simulink model "MOIsolatedBuck2"  (R2013a)
settings: Solver=ode45  StartTime=0.0  StopTime=0.25  RelTol=1e-3
libraries: powerlib x27
settings Model: Creator=Sony  LastModifiedBy=Yooshaa

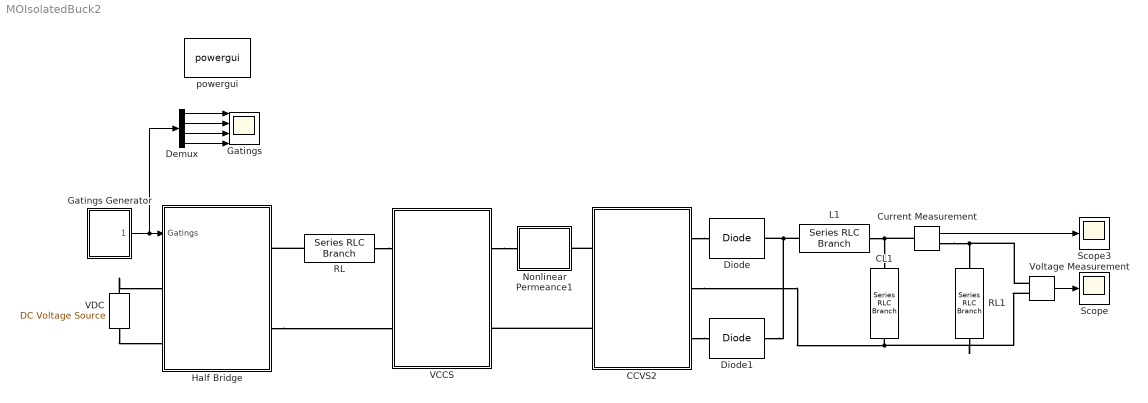
== system MOIsolatedBuck2 ==
  CCVS2 : Subsystem  mask{N=1}
  CL1 : powerlib/Elements/Series RLC Branch  LConnTagsString=__new0  RConnTagsString=__new0  BranchType=C  Resistance=1  Inductance=1e-3  SetiL0=off  InitialCurrent=0  Capacitance=1e-9  Setx0=off  InitialVoltage=0  Measurements=None
  Current Measurement : powerlib/Measurements/Current Measurement  PhasorSimulation=off  OutputType=Complex  PSBequivalent=0
  Demux : Demux
  Diode : powerlib/Power Electronics/Diode  Ron=1e-3  Lon=0  Vf=2  IC=0  UseSnubber=off  Rs=500  Cs=250e-9  Measurements=off
  Diode1 : powerlib/Power Electronics/Diode  Ron=1e-3  Lon=0  Vf=2  IC=0  UseSnubber=off  Rs=500  Cs=250e-9  Measurements=off
  Gatings : Scope  NumInputPorts=4
      settings: YMin=-1~-1~-1~-1  YMax=2~2~2~2  SaveName=ScopeData2
  Gatings Generator : Subsystem  mask{Fs=150000, D=75}
  Half Bridge : Subsystem
  L1 : powerlib/Elements/Series RLC Branch  LConnTagsString=__new0  RConnTagsString=__new0  BranchType=L  Resistance=1  Inductance=.17e-5  SetiL0=off  InitialCurrent=0  Capacitance=1e-6  Setx0=off  InitialVoltage=0  Measurements=None
  Nonlinear Permeance1 : Subsystem  mask{R=1e9, C=3.8e-5, Rm=8}
  RL : powerlib/Elements/Series RLC Branch  LConnTagsString=__new0  RConnTagsString=__new0  BranchType=RL  Resistance=1  Inductance=1e-5  SetiL0=off  InitialCurrent=0  Capacitance=1e-6  Setx0=off  InitialVoltage=0  Measurements=None
  RL1 : powerlib/Elements/Series RLC Branch  LConnTagsString=__new0  RConnTagsString=__new0  BranchType=R  Resistance=1/20  Inductance=1e-3  SetiL0=off  InitialCurrent=0  Capacitance=1e-6  Setx0=off  InitialVoltage=0  Measurements=None
  Scope : Scope
      settings: YMin=4.675  YMax=5.175  SaveName=Vou
  Scope3 : Scope
      settings: YMin=45  YMax=105  SaveName=Iou
  VCCS : Subsystem  mask{N=22}
  VDC : powerlib/Electrical Sources/DC Voltage Source  Amplitude=160  Measurements=None
  Voltage Measurement : powerlib/Measurements/Voltage Measurement  PhasorSimulation=off  OutputType=Complex  PSBequivalent=0
  powergui : powerlib/powergui  Priority=1  SimulationMode=Discrete  SolverType=Backward Euler  SampleTime=1e-7  frequency=60  SPID=on  DisableSnubberDevices=off  DisableRonSwitches=off  DisableVfSwitches=off  SwTol=0  Interpol=off  DisplayEquations=off  frequencyindice=0  Pbase=100e6  ErrMax=1e-4  Iterations=50  UnitsV=kV  UnitsW=MW  FunctionMessages=off  echomessages=off  HookPort=off  EnableUseOfTLC=off  x0status=blocks  RestoreLinks=warning  ResistiveCurrentMeasurement=off  Frange=[0:2:500]  Ylog=off  Xlog=on  ShowGrid=off  save=off  variable=ZData  ZoomFFT=off  StartTime=0.0  cycles=1  DisplayStyle=1  fundamental=60  FreqAxis=off  MaxFrequency=1000  frequencyindicesteady=1  RmsSteady=1  display=off  Ts=0  methode=off
  wires:
  Gatings Generator/1(Gatings) -> Demux/1, Half Bridge/1(Gatings)
  Voltage Measurement/1 -> Scope/1
  Current Measurement/1 -> Scope3/1
  Demux/1 -> Gatings/1
  Demux/2 -> Gatings/2
  Demux/3 -> Gatings/3
  Demux/4 -> Gatings/4
  connections:
  VDC/RConn1 -- Half Bridge/LConn1
  VDC/LConn1 -- Half Bridge/LConn2
  RL/LConn1 -- Half Bridge/RConn1
  Half Bridge/RConn2 -- VCCS/LConn2
  CCVS2/RConn1 -- Diode/LConn1
  CCVS2/RConn3 -- Diode1/LConn1
  CCVS2/RConn2 -- Voltage Measurement/LConn2 -- RL1/LConn1 -- CL1/LConn1
  VCCS/RConn1 -- Nonlinear Permeance1/LConn1
  Diode1/RConn1 -- L1/RConn1 -- Diode/RConn1
  Voltage Measurement/LConn1 -- Current Measurement/RConn1 -- RL1/RConn1
  RL/RConn1 -- VCCS/LConn1
  CCVS2/LConn1 -- Nonlinear Permeance1/RConn1
  Current Measurement/LConn1 -- L1/LConn1 -- CL1/RConn1
  CCVS2/LConn2 -- VCCS/RConn2

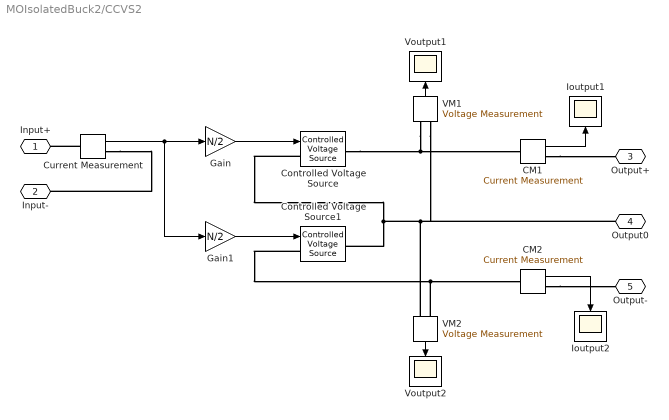
== system MOIsolatedBuck2/CCVS2 ==
  CM1 : powerlib/Measurements/Current Measurement  PhasorSimulation=off  OutputType=Complex  PSBequivalent=0
  CM2 : powerlib/Measurements/Current Measurement  PhasorSimulation=off  OutputType=Complex  PSBequivalent=0
  Controlled Voltage Source : powerlib/Electrical Sources/Controlled Voltage Source  Initialize=on  Source_Type=AC  Amplitude=0  Phase=0  Frequency=0  Measurements=None
  Controlled Voltage Source1 : powerlib/Electrical Sources/Controlled Voltage Source  Initialize=on  Source_Type=AC  Amplitude=0  Phase=0  Frequency=0  Measurements=None
  Current Measurement : powerlib/Measurements/Current Measurement  PhasorSimulation=off  OutputType=Complex  PSBequivalent=0
  Gain : Gain  Gain=N/2
  Gain1 : Gain  Gain=N/2
  Ioutput1 : Scope
      settings: YMin=-2e+10  YMax=2e+10  SaveName=Ioup
  Ioutput2 : Scope
      settings: YMin=-10  YMax=150  SaveName=Ioun
  VM1 : powerlib/Measurements/Voltage Measurement  PhasorSimulation=off  OutputType=Complex  PSBequivalent=0
  VM2 : powerlib/Measurements/Voltage Measurement  PhasorSimulation=off  OutputType=Complex  PSBequivalent=0
  Voutput1 : Scope
      settings: YMin=-2.25e+11  YMax=2.25e+11  SaveName=Voup
  Voutput2 : Scope
      settings: YMin=-20  YMax=20  SaveName=Voun
  Input+ : PMIOPort  Port=1  Side=Left
  Input- : PMIOPort  Port=2  Side=Left
  Output+ : PMIOPort  Port=3  Side=Right
  Output0 : PMIOPort  Port=4  Side=Right
  Output- : PMIOPort  Port=5  Side=Right
  wires:
  Gain/1 -> Controlled Voltage Source/1
  Current Measurement/1 -> Gain1/1, Gain/1
  Gain1/1 -> Controlled Voltage Source1/1
  VM2/1 -> Voutput2/1
  VM1/1 -> Voutput1/1
  CM2/1 -> Ioutput2/1
  CM1/1 -> Ioutput1/1
  connections:
  Current Measurement/LConn1 -- Input+/RConn1
  Current Measurement/RConn1 -- Input-/RConn1
  Controlled Voltage Source/RConn1 -- CM1/LConn1 -- VM1/LConn1
  Controlled Voltage Source/LConn1 -- Output0/RConn1 -- VM1/LConn2 -- VM2/LConn1 -- Controlled Voltage Source1/RConn1
  Controlled Voltage Source1/LConn1 -- VM2/LConn2 -- CM2/LConn1
  CM1/RConn1 -- Output+/RConn1
  CM2/RConn1 -- Output-/RConn1

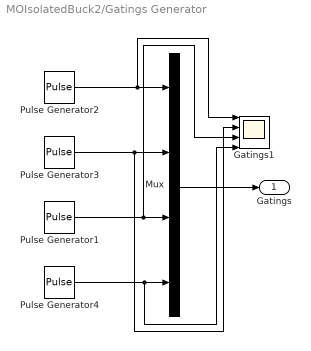
== system MOIsolatedBuck2/Gatings Generator ==
  Gatings1 : Scope  NumInputPorts=4
      settings: YMin=-1~-1~-1~-1  YMax=2~2~2~2  SaveName=ScopeData3
  Mux : Mux
  Pulse Generator1 : DiscretePulseGenerator  PulseType=Time based  Period=2/Fs  PulseWidth=50  PhaseDelay=(1/Fs)
  Pulse Generator2 : DiscretePulseGenerator  PulseType=Time based  Period=2/Fs  PulseWidth=50  PhaseDelay=-((100-D)/100)*(1/Fs)
  Pulse Generator3 : DiscretePulseGenerator  PulseType=Time based  Period=2/Fs  PulseWidth=50  PhaseDelay=(D/100)*(1/Fs)
  Pulse Generator4 : DiscretePulseGenerator  PulseType=Time based  Period=2/Fs  PulseWidth=50
  Gatings : Outport
  wires:
  Mux/1 -> Gatings/1
  Pulse Generator2/1 -> Gatings1/1, Mux/1
  Pulse Generator1/1 -> Gatings1/3, Mux/3
  Pulse Generator3/1 -> Gatings1/2, Mux/2
  Pulse Generator4/1 -> Gatings1/4, Mux/4

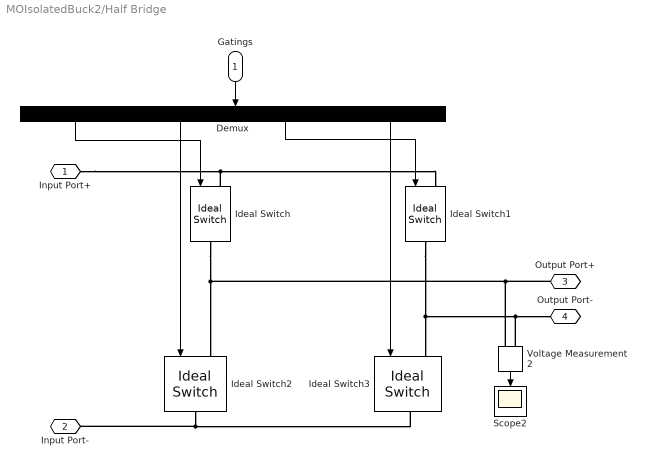
== system MOIsolatedBuck2/Half Bridge ==
  Gatings : Inport
  Demux : Demux
  Ideal Switch{,1..3} (4 alike) : powerlib/Power Electronics/Ideal Switch  Ron=0.001  Lon=0  IC=0  Rs=1e5  Cs=inf  Measurements=off
  Scope2 : Scope
      settings: YMin=-175  YMax=175  SaveName=Vinput
  Voltage Measurement2 : powerlib/Measurements/Voltage Measurement  PhasorSimulation=off  OutputType=Complex  PSBequivalent=0
  Input Port+ : PMIOPort  Port=1  Side=Left
  Input Port- : PMIOPort  Port=2  Side=Left
  Output Port+ : PMIOPort  Port=3  Side=Right
  Output Port- : PMIOPort  Port=4  Side=Right
  wires:
  Demux/3 -> Ideal Switch1/1
  Demux/1 -> Ideal Switch/1
  Demux/2 -> Ideal Switch2/1
  Gatings/1 -> Demux/1
  Demux/4 -> Ideal Switch3/1
  Voltage Measurement2/1 -> Scope2/1
  connections:
  Ideal Switch/LConn1 -- Ideal Switch1/LConn1 -- Input Port+/RConn1
  Ideal Switch2/RConn1 -- Ideal Switch3/RConn1 -- Input Port-/RConn1
  Ideal Switch1/RConn1 -- Ideal Switch3/LConn1 -- Voltage Measurement2/LConn2 -- Output Port-/RConn1
  Ideal Switch/RConn1 -- Voltage Measurement2/LConn1 -- Output Port+/RConn1 -- Ideal Switch2/LConn1

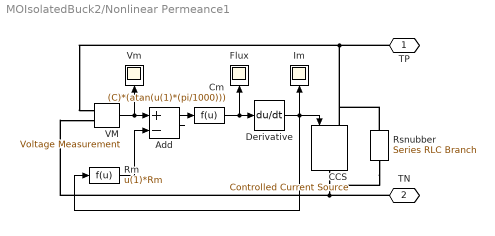
== system MOIsolatedBuck2/Nonlinear Permeance1 ==
  Add : Sum  Inputs=+-
  CCS : powerlib/Electrical Sources/Controlled Current Source  Initialize=on  Source_Type=AC  Amplitude=0  Phase=0  Frequency=0  Measurements=None
  Cm : Fcn  Expr=(C)*(atan(u(1)*(pi/1000)))
  Derivative : Derivative
  Flux : Scope
      settings: YMin=-4e-05  YMax=4e-05  SaveName=PermeanceFlux
  Im : Scope
      settings: TimeRange=0.02  YMin=-200  YMax=200  SaveName=PermeanceIm
  Rm : Fcn  Expr=u(1)*Rm
  Rsnubber : powerlib/Elements/Series RLC Branch  LConnTagsString=__new0  RConnTagsString=__new0  BranchType=R  Resistance=R  Inductance=1e-3  SetiL0=off  InitialCurrent=0  Capacitance=1e-6  Setx0=off  InitialVoltage=0  Measurements=None
  VM : powerlib/Measurements/Voltage Measurement  PhasorSimulation=off  OutputType=Complex  PSBequivalent=0
  Vm : Scope
      settings: YMin=-4000  YMax=4000  SaveName=PermeanceVm
  TP : PMIOPort  Port=1  Side=Left
  TN : PMIOPort  Port=2  Side=Right
  wires:
  VM/1 -> Add/1, Vm/1
  Cm/1 -> Flux/1, Derivative/1
  Rm/1 -> Add/2
  Derivative/1 -> Rm/1, CCS/1, Im/1
  Add/1 -> Cm/1
  connections:
  TN/RConn1 -- Rsnubber/RConn1 -- CCS/RConn1 -- VM/LConn2
  TP/RConn1 -- Rsnubber/LConn1 -- CCS/LConn1 -- VM/LConn1

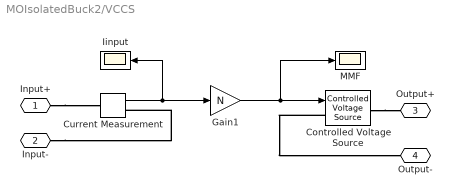
== system MOIsolatedBuck2/VCCS ==
  Controlled Voltage Source : powerlib/Electrical Sources/Controlled Voltage Source  Initialize=off  Source_Type=AC  Amplitude=0  Phase=0  Frequency=0  Measurements=None
  Current Measurement : powerlib/Measurements/Current Measurement  PhasorSimulation=off  OutputType=Complex  PSBequivalent=0
  Gain1 : Gain  Gain=N
  Iinput : Scope
      settings: YMin=0  YMax=150  SaveName=Iprimary
  MMF : Scope
      settings: YMin=0  YMax=15000  SaveName=MMF
  Input+ : PMIOPort  Port=1  Side=Left
  Input- : PMIOPort  Port=2  Side=Left
  Output+ : PMIOPort  Port=3  Side=Right
  Output- : PMIOPort  Port=4  Side=Right
  wires:
  Current Measurement/1 -> Iinput/1, Gain1/1
  Gain1/1 -> MMF/1, Controlled Voltage Source/1
  connections:
  Input+/RConn1 -- Current Measurement/LConn1
  Input-/RConn1 -- Current Measurement/RConn1
  Controlled Voltage Source/RConn1 -- Output+/RConn1
  Controlled Voltage Source/LConn1 -- Output-/RConn1
